simulink model "testNullstellesim"  (Simulink 7.9)
settings: Solver=ode45  StartTime=0.0  StopTime=10.0  RelTol=1e-3
values from neighbouring files (symbols this model uses):
  A = [1 0; 0 1]    [testDifferenzordnung.m]
  B = [1 0]'    [testDifferenzordnung.m]
  C = [0 1]    [testDifferenzordnung.m]
  D = 0    [testDifferenzordnung.m]
undefined symbols (not defined in the file or in its folder): nst, u0, x0
settings Model: Creator=BPeixoto  LastModifiedBy=BPeixoto

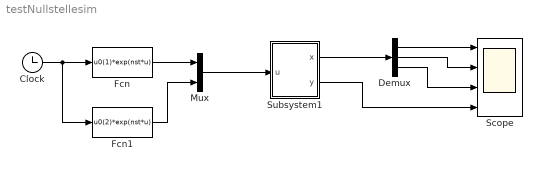
== system testNullstellesim ==
  Clock : Clock
  Demux : Demux  Outputs=3
  Fcn : Fcn  Expr=u0(1)*exp(nst*u)
  Fcn1 : Fcn  Expr=u0(2)*exp(nst*u)
  Mux : Mux  Inputs=2
  Scope : Scope  NumInputPorts=4
      settings: YMin=-5~-5~-5~-5  YMax=5~5~5~5
  Subsystem1 : Subsystem
  wires:
  Clock/1 -> Fcn/1, Fcn1/1
  Fcn1/1 -> Mux/2
  Fcn/1 -> Mux/1
  Mux/1 -> Subsystem1/1(u)
  Subsystem1/2(y) -> Scope/4
  Subsystem1/1(x) -> Demux/1
  Demux/1 -> Scope/1
  Demux/2 -> Scope/2
  Demux/3 -> Scope/3

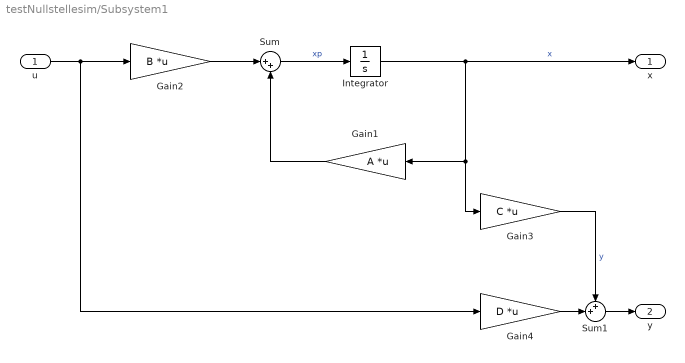
== system testNullstellesim/Subsystem1 ==
  u : Inport
  Gain1 : Gain  Gain=A  Multiplication=Matrix(K*u) (u vector)
  Gain2 : Gain  Gain=B  Multiplication=Matrix(K*u) (u vector)
  Gain3 : Gain  Gain=C  Multiplication=Matrix(K*u) (u vector)
  Gain4 : Gain  Gain=D  Multiplication=Matrix(K*u) (u vector)
  Integrator : Integrator  InitialCondition=x0
  Sum : Sum  Inputs=|++
  Sum1 : Sum  Inputs=++|
  x : Outport
  y : Outport  Port=2
  wires:
  Integrator/1 -> x/1, Gain1/1, Gain3/1  "x"
  Sum/1 -> Integrator/1  "xp"
  Gain1/1 -> Sum/2
  Gain2/1 -> Sum/1
  u/1 -> Gain2/1, Gain4/1
  Gain3/1 -> Sum1/1  "y"
  Sum1/1 -> y/1
  Gain4/1 -> Sum1/2
